simulink model "lab1v2"  (R2013a)
settings: Solver=ode5  StartTime=0.0  StopTime=inf  RelTol=1e-3
undefined symbols (not defined in the file or in its folder): National_Instruments, PCI
libraries: rtwinlib x2
settings Model: Creator=u_labelectro  LastModifiedBy=u_labelectro

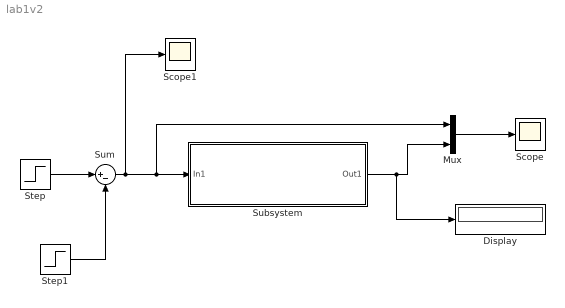
== system lab1v2 ==
  Display : Display
  Mux : Mux  Inputs=2
  Scope : Scope
      settings: YMin=10  YMax=80  SampleInput=on
  Scope1 : Scope
      settings: YMin=20  YMax=20  SampleInput=on
  Step : Step  Time=5  Before=20  After=80
  Step1 : Step  Time=5.1  After=60
  Subsystem : Subsystem
  Sum : Sum  Inputs=|+-
  wires:
  Subsystem/1(Out1) -> Display/1, Mux/2
  Mux/1 -> Scope/1
  Step1/1 -> Sum/2
  Step/1 -> Sum/1
  Sum/1 -> Scope1/1, Mux/1, Subsystem/1(In1)

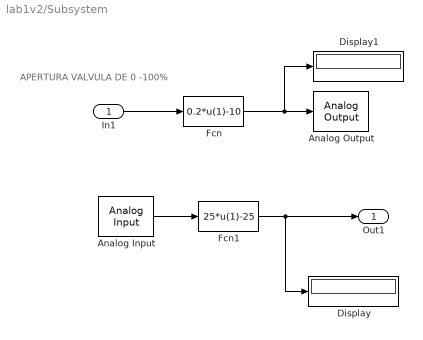
== system lab1v2/Subsystem ==
  note: APERTURA VALVULA DE 0 -100%
  In1 : Inport
  Analog Input : rtwinlib/Analog Input  SampleTime=0.01  MaxMissedTicks=10  ShowMissedTicks=off  YieldWhenWaiting=off  DrvName=National_Instruments/PCI-6229  DrvAddress=4294967295  DrvOptions=[0 0 0 0 0]  Channels=1  RangeMode=1  VoltRange=1  DataType=1
      settings: AttributesFormatString=National Instruments\nPCI-6229 [auto]
  Analog Output : rtwinlib/Analog Output  SampleTime=0.01  MaxMissedTicks=10  ShowMissedTicks=off  YieldWhenWaiting=off  DrvName=National_Instruments/PCI-6229  DrvAddress=4294967295  DrvOptions=[0 0 0 0 0]  Channels=1  RangeMode=1  VoltRange=1  InitialValue=[]  FinalValue=[]
      settings: AttributesFormatString=National Instruments\nPCI-6229 [auto]
  Display : Display
  Display1 : Display
  Fcn : Fcn  Expr=0.2*u(1)-10
  Fcn1 : Fcn  Expr=25*u(1)-25
  Out1 : Outport
  wires:
  In1/1 -> Fcn/1
  Fcn/1 -> Display1/1, Analog Output/1
  Analog Input/1 -> Fcn1/1
  Fcn1/1 -> Out1/1, Display/1
